simulink model "InvertedDoublePendulumOnCart"  (R2016a)
settings: Solver=VariableStepAuto  StartTime=0.0  StopTime=10.0  RelTol=1e-3
values from neighbouring files (symbols this model uses):
  b0 = 0.15    [PendulumParameter.m]    (also in PendulumParameterT.m)
  b1 = 0.005    [PendulumParameter.m]    (also in PendulumParameter1.m; PendulumParameterT.m)
  b2 = 0.005    [PendulumParameter.m]    (also in PendulumParameter1.m; PendulumParameterT.m)
  g = 9.81    [LQRControllerPrevious.m]    (also in PendulumParameter.m; PendulumParameter1.m)
  I1 = I10+m1*(R1^2)    (= 0.00365625)    [LQRControllerPrevious.m]    (also in PendulumParameter.m = 0.624; PendulumParameter1.m = 0.624; PendulumParameterT.m)
  I2 = I20+m2*(R2^2)    (= 0.00325)    [LQRControllerPrevious.m]    (also in PendulumParameter.m = 0.624; PendulumParameter1.m = 0.624; PendulumParameterT.m)
  L1 = 0.15    [LQRControllerPrevious.m]    (also in PendulumParameter.m = 2.4; PendulumParameter1.m = 2.4; PendulumParameterT.m)
  L2 = 0.2    [LQRControllerPrevious.m]    (also in PendulumParameter.m = 2.4; PendulumParameter1.m = 2.4; PendulumParameterT.m)
  m0 = 0.67    [LQRControllerPrevious.m]    (also in PendulumParameter.m = 5; PendulumParameterT.m)
  m1 = 0.15    [LQRControllerPrevious.m]    (also in PendulumParameter.m = 0.1; PendulumParameter1.m = 0.1; PendulumParameterT.m)
  m2 = 0.075    [LQRControllerPrevious.m]    (also in PendulumParameter.m = 0.1; PendulumParameter1.m = 0.1; PendulumParameterT.m)
  theta1 = 0    [PendulumParameter.m]    (also in PendulumParameter1.m; PendulumParameterT.m)
  theta2 = 0    [PendulumParameter.m]    (also in PendulumParameter1.m; PendulumParameterT.m)
  xx = 0    [PendulumParameter.m]    (also in PendulumParameter1.m; PendulumParameterT.m)
settings Model: Creator=VAIO  LastModifiedBy=VAIO
settings DebuggingCC: InitInArrayFormatMsg=none

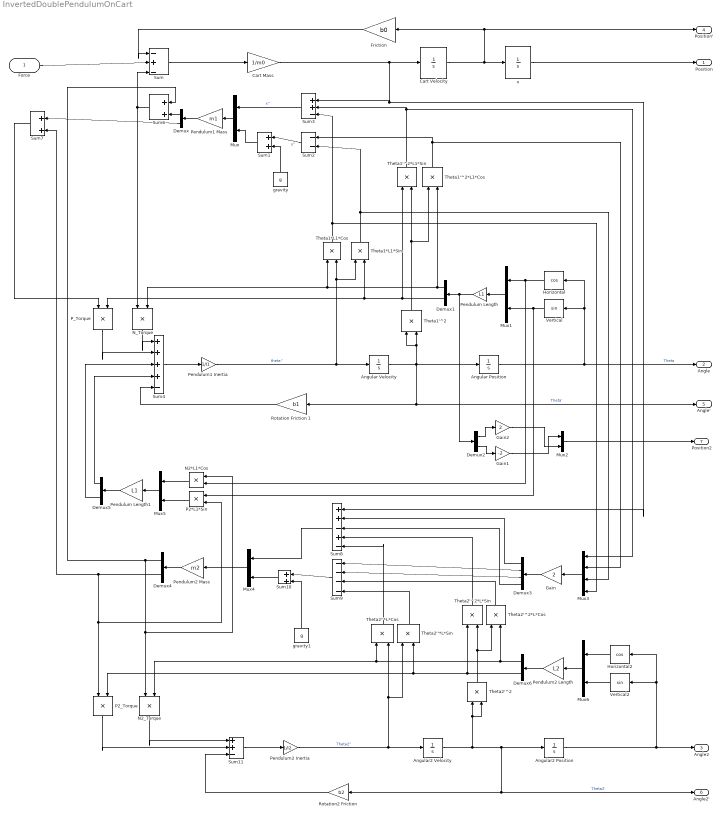
== system InvertedDoublePendulumOnCart ==
  "Force " : Inport
  "  Vertical" : Trigonometry  NumberOfIterations=15
  "  Vertical2" : Trigonometry  NumberOfIterations=15
  Angular Velocity : Integrator
  Angular Position : Integrator  InitialCondition=theta1
  Angular2 Position : Integrator  InitialCondition=theta2
  Angular2 Velocity : Integrator
  Cart Velocity : Integrator
  Cart Mass : Gain  Gain=1/m0
  Demux{,1..2,4..6} (6 alike) : Demux  Outputs=2
  Demux3 : Demux
  Friction : Gain  Gain=b0
  Gain : Gain  Gain=2
  Gain1 : Gain  Gain=-2
  Gain2 : Gain  Gain=2
  "Horizontal  " : Trigonometry  Operator=cos  NumberOfIterations=15
  Horizontal2 : Trigonometry  Operator=cos  NumberOfIterations=15
  Mux{,1..2,4..6} (6 alike) : Mux  Inputs=2
  Mux3 : Mux
  N2*L1*Cos : Product
  N2_Torque : Product
  N_Torque : Product
  P2*L1*Sin : Product
  P2_Torque : Product
  P_Torque : Product
  Pendulum Length1 : Gain  Gain=L1
  Pendulum Length : Gain  Gain=L1
  Pendulum1 Mass : Gain  Gain=m1
  Pendulum1 Inertia : Gain  Gain=1/I1
  Pendulum2 Length : Gain  Gain=L2
  Pendulum2 Mass : Gain  Gain=m2
  Pendulum2 Inertia : Gain  Gain=1/I2
  Rotation Friction 1 : Gain  Gain=b1
  Rotation2 Friction : Gain  Gain=b2
  Sum : Sum  Inputs=|-+-
  Sum{1,6..7,10} (4 alike) : Sum  Inputs=|++
  Sum11 : Sum  Inputs=|++-
  Sum2 : Sum  Inputs=|--
  Sum3 : Sum  Inputs=|++-
  Sum4 : Sum  Inputs=|++++-
  Sum8 : Sum  Inputs=|++-+-
  Sum9 : Sum  Inputs=|----
  Theta1'^2 : Product
  Theta1'^2*L1*Cos : Product
  Theta1'^2*L1*Sin : Product
  Theta1*L1*Cos : Product
  Theta1*L1*Sin : Product
  Theta2''*L*Cos : Product
  Theta2''*L*Sin : Product
  Theta2'^2 : Product
  Theta2'^2*L*Cos : Product
  Theta2'^2*L*Sin : Product
  gravity : Constant  Value=g
  gravity1 : Constant  Value=g
  x : Integrator  InitialCondition=xx
  Position : Outport
  Angle : Outport  Port=2
  Angle2 : Outport  Port=3
  Position' : Outport  Port=4
  Angle' : Outport  Port=5
  Angle2' : Outport  Port=6
  Position2 : Outport  Port=7
  wires:
  "Force "/1 -> Sum/2
  Sum/1 -> Cart Mass/1
  Cart Velocity/1 -> Friction/1, Position'/1, x/1
  x/1 -> Position/1
  Friction/1 -> Sum/1
  Pendulum1 Mass/1 -> Demux/1
  Mux/1 -> Pendulum1 Mass/1
  Sum1/1 -> Mux/2
  gravity/1 -> Sum1/2
  Sum2/1 -> Sum1/1  "y''"
  Sum3/1 -> Mux/1  "x''"
  Mux1/1 -> Pendulum Length/1
  "  Vertical"/1 -> P2*L1*Sin/1, Mux1/2
  "Horizontal  "/1 -> Mux1/1, N2*L1*Cos/2
  Pendulum Length/1 -> Demux1/1, Demux2/1
  Sum4/1 -> Pendulum1 Inertia/1
  Pendulum1 Inertia/1 -> Theta1*L1*Sin/1, Theta1*L1*Cos/2, Angular Velocity/1  "theta''"
  Angular Velocity/1 -> Theta1'^2/1, Theta1'^2/2, Angular Position/1, Rotation Friction 1/1, Angle'/1  "Theta'"
  Angular Position/1 -> "Horizontal  "/1, "  Vertical"/1, Angle/1  "Theta"
  Rotation Friction 1/1 -> Sum4/5
  Demux2/2 -> Gain1/1
  Demux2/1 -> Gain2/1
  Gain2/1 -> Mux2/2
  Gain1/1 -> Mux2/1
  Mux2/1 -> Position2/1
  N_Torque/1 -> Sum4/1
  P_Torque/1 -> Sum4/2
  Demux1/2 -> Theta1'^2*L1*Sin/1, P_Torque/2, Theta1*L1*Sin/2
  Demux1/1 -> N_Torque/2, Theta1*L1*Cos/1, Theta1'^2*L1*Cos/2
  Demux/1 -> Sum6/2
  Sum6/1 -> N_Torque/1, Sum/3
  Demux/2 -> Sum7/1
  Sum7/1 -> P_Torque/1
  Mux3/1 -> Gain/1
  Cart Mass/1 -> Sum8/1, Sum3/1, Cart Velocity/1
  Theta1'^2*L1*Sin/1 -> Mux3/1, Sum3/2
  Theta1'^2*L1*Cos/1 -> Sum2/1, Mux3/2
  Theta1*L1*Sin/1 -> Sum2/2, Mux3/3
  Theta1*L1*Cos/1 -> Mux3/4, Sum3/3
  Gain/1 -> Demux3/1
  Demux3/2 -> Sum9/1
  Demux3/3 -> Sum9/2
  Demux3/4 -> Sum8/3
  Demux3/1 -> Sum8/2
  Sum9/1 -> Sum10/1
  gravity1/1 -> Sum10/2
  Sum10/1 -> Mux4/2
  Sum8/1 -> Mux4/1
  Mux4/1 -> Pendulum2 Mass/1
  Pendulum2 Mass/1 -> Demux4/1
  Demux4/1 -> N2*L1*Cos/1, N2_Torque/1, Sum6/1
  Mux5/1 -> Pendulum Length1/1
  Pendulum Length1/1 -> Demux5/1
  P2*L1*Sin/1 -> Mux5/2
  N2*L1*Cos/1 -> Mux5/1
  Demux5/1 -> Sum4/4
  Demux5/2 -> Sum4/3
  Horizontal2/1 -> Mux6/1
  "  Vertical2"/1 -> Mux6/2
  Mux6/1 -> Pendulum2 Length/1
  Pendulum2 Length/1 -> Demux6/1
  Angular2 Position/1 -> "  Vertical2"/1, Horizontal2/1, Angle2/1
  Angular2 Velocity/1 -> Theta2'^2/2, Theta2'^2/1, Angle2'/1, Rotation2 Friction/1, Angular2 Position/1  "Theta2'"
  Pendulum2 Inertia/1 -> Theta2''*L*Sin/1, Theta2''*L*Cos/2, Angular2 Velocity/1  "Theta2''"
  Sum11/1 -> Pendulum2 Inertia/1
  Rotation2 Friction/1 -> Sum11/3
  N2_Torque/1 -> Sum11/1
  P2_Torque/1 -> Sum11/2
  Demux6/2 -> Theta2'^2*L*Sin/1, P2_Torque/2, Theta2''*L*Sin/2
  Demux6/1 -> N2_Torque/2, Theta2''*L*Cos/1, Theta2'^2*L*Cos/2
  Theta2'^2/1 -> Theta2'^2*L*Cos/1, Theta2'^2*L*Sin/2
  Theta2'^2*L*Cos/1 -> Sum9/3
  Theta2'^2*L*Sin/1 -> Sum8/4
  Theta2''*L*Sin/1 -> Sum9/4
  Theta2''*L*Cos/1 -> Sum8/5
  Demux4/2 -> P2*L1*Sin/2, P2_Torque/1, Sum7/2
  Theta1'^2/1 -> Theta1'^2*L1*Cos/1, Theta1'^2*L1*Sin/2
